simulink model "EngineModel_scaled_27_7_2016_with_new_maps"  (R2021a)
settings: Solver=ode4  StartTime=0.0  StopTime=30  FixedStep=0.2  RelTol=1e-3  EnableMultiTasking=on
values from neighbouring files (symbols this model uses):
  Fanmap_2 = [1 1 1 1 1 1 1 1 1 1 275.724 325.4224 ... (330 elements, 10x3x11)]    [enginemaps2.mat]
  HPCompmap_2 = [1 1 1 1 1 1 1 1 1 1 32.390865 37.6623195 ... (330 elements, 10x3x11)]    [enginemaps2.mat]
  HPTurbinemap_2 = [0.24979968 0.24979968 0.24979968 0.24979968 0.24979968 0.24979968 0.24979968 0.24979968 0.24979968 0.24979968 0.004250667 0.005047667 ... (330 elements, 10x3x11)]    [enginemaps2.mat]
  LPCompmap_2 = [1 1 1 1 1 1 1 1 1 1 34.17260994 40.23277722 ... (330 elements, 10x3x11)]    [enginemaps2.mat]
  LPTurbinemap_2 = [0.665969797 0.665969797 0.665969797 0.665969797 0.665969797 0.665969797 0.665969797 0.665969797 0.00912 0.013173333 0.015706667 0.01672 ... (264 elements, 8x3x11)]    [enginemaps2.mat]
undefined symbols (not defined in the file or in its folder): Adiabatic_compression_fan, Adiabatic_compression_HPC, Adiabatic_compression_LPC, coldnozzle, compression_ram, cond_f2, D, datatables, hotnozzle, HPT1, if_Nth, if_Ntl, if_Z, LPT, performance1, thermo_combustor, turbo
libraries: dspmtrx3 x10, aerolibatmos2 x8, dspsigattribs x3, dspsolvers x2, dspfactors x1
(part 1 of 14)
settings Model: Creator=BES  LastModifiedBy=PhD
settings SolverCC: ZeroCrossAlgorithm=Adaptive  AlgebraicLoopSolver=TrustRegion
settings DataIOCC: InitialState=load('enginemaps1.mat')  SaveFormat=Array  ReturnWorkspaceOutputs=off
settings OptimizationCC: LifeSpan=inf
settings DebuggingCC: UnderspecifiedInitializationDetection=Classic  MergeDetectMultiDrivingBlocksExec=none  SolverPrmCheckMsg=warning  StateNameClashWarn=warning  SFUnexpectedBacktrackingDiag=warning  SFNoUnconditionalDefaultTransitionDiag=warning  SFExecutionAtInitializationDiag=none  SFMachineParentedDataDiag=warning  ArithmeticOperatorsInVariantConditions=warning
settings HardwareCC: ProdBitPerPointer=32  ProdBitPerSizeT=32  ProdBitPerPtrDiffT=32  ProdLargestAtomicFloat=None  ProdIntDivRoundTo=Undefined  ProdEndianess=Unspecified  ProdWordSize=32  ProdHWDeviceType=32-bit Generic
settings ModelReferenceCC: PropagateSignalLabelsOutOfModel=off
settings SFSimCC: SimUseLocalCustomCode=off  CustomCodeUndefinedFunction=UseInterfaceOnly
settings RTWCC: RTWUseLocalCustomCode=off
settings CodeAppCC: StateflowObjectComments=on
settings GRTTargetCC: TargetLangStandard=C89/C90 (ANSI)
settings ConfigComp: CovMetricSettings=dw  CovSaveCumulativeToWorkspaceVar=on  CovSaveSingleToWorkspaceVar=on  CovExternalEMLEnable=off
settings SimscapeCC: SimscapeNormalizeSystem=off
settings ConfigurationSet: Description=SimMechanics 2G

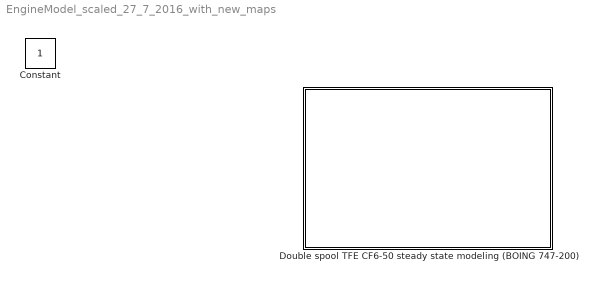
== system EngineModel_scaled_27_7_2016_with_new_maps ==
  Double spool TFE CF6-50 steady state modeling (BOING 747-200) : Subsystem
      mask Display: image('b747.jpg')
  Constant : Constant  IOType=siggen

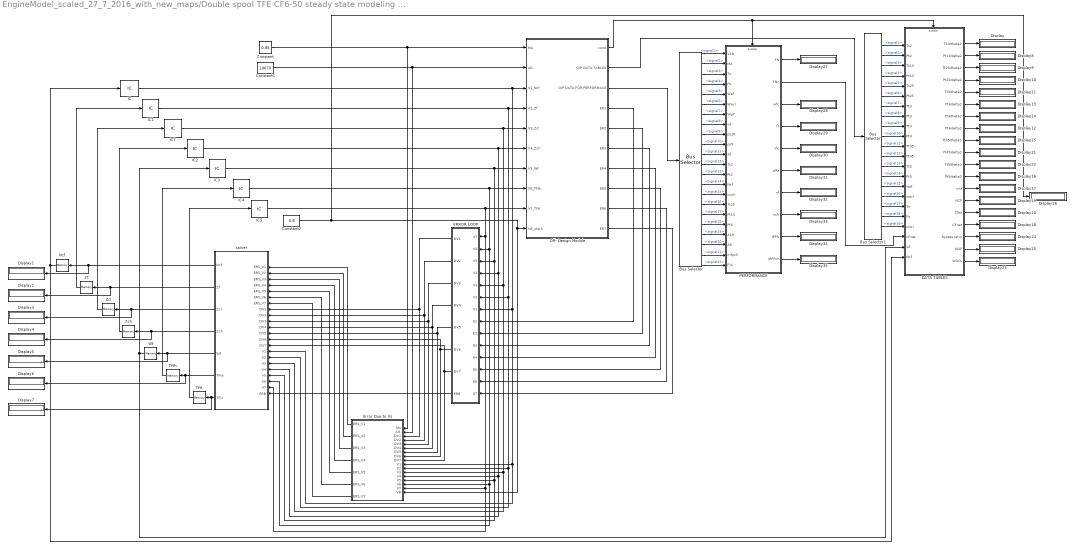
== system EngineModel_scaled_27_7_2016_with_new_maps/Double spool TFE CF6-50 steady state modeling (BOING 747-200) ==
  Bus Selector : BusSelector  OutputSignals=signal1,signal2,signal3,signal4,signal5,signal6,signal7,signal8,signal9,signal10,signal11,signal12,signal13,signal14,signal15,signal16,signal17,signal18,signal19,signal20,signal21,signal22
  Bus Selector1 : BusSelector  OutputSignals=signal1,signal2,signal3,signal4,signal5,signal6,signal7,signal8,signal9,signal10,signal11,signal12,signal13,signal14,signal15,signal16,signal17,signal18,signal19
  Constant : Constant  Value=0.85
  Constant1 : Constant  Value=10670
  Constant2 : Constant  Value=0.8  VectorParams1D=off
  DATA TABLES : Subsystem
  Display{,1..35} (36 alike) : Display
  "ERROR LOOP " : Subsystem
  Error Due to Vs : Subsystem
  IC : InitialCondition
  IC1 : InitialCondition  Value=0.83333
  IC2 : InitialCondition  Value=0.83333
  IC3 : InitialCondition  Value=0.89
  IC4 : InitialCondition  Value=156
  IC5 : InitialCondition  Value=674
  IC7 : InitialCondition  Value=0.83333
  Ncf : Memory  InitialCondition=1
  Off- Design Module : Subsystem
  PERFORMANCE : Subsystem
  TFth : Memory  InitialCondition=156
  TFtl : Memory  InitialCondition=674
  Wf : Memory  InitialCondition=0.89
  Zch : Memory  InitialCondition=0.83333
  Zcl : Memory  InitialCondition=0.83333
  Zf : Memory  InitialCondition=0.83333
  solver : Subsystem
  wires:
  Constant/1 -> Error Due to Vs/1(Mo), Off- Design Module/1(Mo)
  Constant1/1 -> Error Due to Vs/2(Alt.), Off- Design Module/2(Alt.)
  "ERROR LOOP "/1(DV1) -> solver/8(DV1), Error Due to Vs/3(DV1)
  "ERROR LOOP "/2(DV2) -> solver/9(DV2), Error Due to Vs/4(DV2)
  "ERROR LOOP "/3(DV3) -> solver/10(DV3), Error Due to Vs/5(DV3)
  "ERROR LOOP "/4(DV4) -> solver/11(DV4), Error Due to Vs/6(DV4)
  "ERROR LOOP "/5(DV5) -> solver/12(DV5), Error Due to Vs/7(DV5)
  "ERROR LOOP "/6(DV6) -> solver/13(DV6), Error Due to Vs/8(DV6)
  "ERROR LOOP "/7(DV7) -> solver/14(DV7), Error Due to Vs/9(DV7)
  solver/1(Ncf) -> Display1/1, Ncf/1
  solver/2(Zf) -> Zf/1, Display2/1
  solver/3(Zcl) -> Display3/1, Zcl/1
  solver/4(Zch) -> Display4/1, Zch/1
  solver/5(Wf) -> Display5/1, Wf/1
  solver/6(TFth) -> Display6/1, TFth/1
  solver/7(TFtl) -> Display7/1, TFtl/1
  Off- Design Module/4(ER1) -> "ERROR LOOP "/8(E1)
  Off- Design Module/5(ER2) -> "ERROR LOOP "/9(E2)
  Off- Design Module/6(ER3) -> "ERROR LOOP "/10(E3)
  Off- Design Module/7(ER4) -> "ERROR LOOP "/11(E4)
  Off- Design Module/8(ER5) -> "ERROR LOOP "/12(E5)
  Off- Design Module/9(ER6) -> "ERROR LOOP "/13(E6)
  Off- Design Module/10(ER7) -> "ERROR LOOP "/14(E7)
  "ERROR LOOP "/8(ERB) -> solver/22(ERB)
  Error Due to Vs/1(ERS_V1) -> solver/1(ERS_V1)
  Error Due to Vs/2(ERS_V2) -> solver/2(ERS_V2)
  Error Due to Vs/3(ERS_V3) -> solver/3(ERS_V3)
  Error Due to Vs/4(ERS_V4) -> solver/4(ERS_V4)
  Error Due to Vs/5(ERS_V5) -> solver/5(ERS_V5)
  Error Due to Vs/6(ERS_V6) -> solver/6(ERS_V6)
  Error Due to Vs/7(ERS_V7) -> solver/7(ERS_V7)
  IC/1 -> Off- Design Module/3(V1_Ncf), Error Due to Vs/10(V1), solver/15(V1), "ERROR LOOP "/7(V1)
  IC1/1 -> Off- Design Module/4(V2_Zf), solver/16(V2), Error Due to Vs/11(V2), "ERROR LOOP "/6(V2)
  IC7/1 -> Off- Design Module/5(V3_Zcl), "ERROR LOOP "/5(V3), solver/17(V3), Error Due to Vs/12(V3)
  IC2/1 -> solver/18(V4), Error Due to Vs/13(V4), "ERROR LOOP "/4(V4), Off- Design Module/6(V4_Zch)
  IC3/1 -> solver/19(V5), Error Due to Vs/14(V5), "ERROR LOOP "/3(V5), Off- Design Module/7(V5_Wf)
  IC4/1 -> solver/20(V6), Error Due to Vs/15(V6), "ERROR LOOP "/2(V6), Off- Design Module/8(V6_TFth)
  IC5/1 -> Off- Design Module/9(V7_TFtl), solver/21(V7), Error Due to Vs/16(V7), "ERROR LOOP "/1(V7)
  Constant2/1 -> Display26/1, Error Due to Vs/17(VB), Off- Design Module/10(VB_cNch)
  Off- Design Module/3(O/P DATA FOR PERFORMACE) -> Bus Selector/1
  Off- Design Module/1(cond) -> DATA TABLES/Enable, PERFORMANCE/Enable
  Bus Selector/20 -> PERFORMANCE/20(A9)  "<signal20>"
  Bus Selector/19 -> PERFORMANCE/19(A19)  "<signal19>"
  Bus Selector/18 -> PERFORMANCE/18(Pt5)  "<signal18>"
  Bus Selector/17 -> PERFORMANCE/17(Pt13)  "<signal17>"
  Bus Selector/16 -> PERFORMANCE/16(Tt25)  "<signal16>"
  Bus Selector/15 -> PERFORMANCE/15(cnch)  "<signal15>"
  Bus Selector/14 -> PERFORMANCE/14(Ncf)  "<signal14>"
  Bus Selector/13 -> PERFORMANCE/13(Pt2)  "<signal13>"
  Bus Selector/12 -> PERFORMANCE/12(Tt2)  "<signal12>"
  Bus Selector/11 -> PERFORMANCE/11(wf)  "<signal11>"
  Bus Selector/10 -> PERFORMANCE/10(ps9)  "<signal10>"
  Bus Selector/9 -> PERFORMANCE/9(ps10)  "<signal9>"
  Bus Selector/8 -> PERFORMANCE/8(v9)  "<signal8>"
  Bus Selector/7 -> PERFORMANCE/7(Wg7)  "<signal7>"
  Bus Selector/6 -> PERFORMANCE/6(Wacl)  "<signal6>"
  Bus Selector/5 -> PERFORMANCE/5(Waf)  "<signal5>"
  Bus Selector/4 -> PERFORMANCE/4(Po)  "<signal4>"
  Bus Selector/3 -> PERFORMANCE/3(To)  "<signal3>"
  Bus Selector/2 -> PERFORMANCE/2(Mo)  "<signal2>"
  Bus Selector/1 -> PERFORMANCE/1(V19)  "<signal1>"
  TFtl/1 -> IC5/1
  TFth/1 -> IC4/1
  Wf/1 -> DATA TABLES/21(wf), IC3/1
  Zch/1 -> IC2/1
  Zcl/1 -> IC7/1
  Zf/1 -> IC1/1
  Ncf/1 -> DATA TABLES/22(Ncf), IC/1
  Off- Design Module/2(O/P DATA TABLES) -> Bus Selector1/1
  Bus Selector1/1 -> DATA TABLES/1(Tt2)  "<signal1>"
  Bus Selector1/2 -> DATA TABLES/2(Pt2)  "<signal2>"
  Bus Selector1/3 -> DATA TABLES/3(Tt13)  "<signal3>"
  Bus Selector1/4 -> DATA TABLES/4(Pt13)  "<signal4>"
  Bus Selector1/5 -> DATA TABLES/5(Tt25)  "<signal5>"
  Bus Selector1/6 -> DATA TABLES/6(Pt25)  "<signal6>"
  Bus Selector1/7 -> DATA TABLES/7(Tt3)  "<signal7>"
  Bus Selector1/8 -> DATA TABLES/8(Pt3)  "<signal8>"
  Bus Selector1/9 -> DATA TABLES/9(Tt4)  "<signal9>"
  Bus Selector1/10 -> DATA TABLES/10(Pt4)  "<signal10>"
  Bus Selector1/11 -> DATA TABLES/11(Tt45)  "<signal11>"
  Bus Selector1/12 -> DATA TABLES/12(Pt45)  "<signal12>"
  Bus Selector1/13 -> DATA TABLES/13(Tt5)  "<signal13>"
  Bus Selector1/14 -> DATA TABLES/14(Pt5)  "<signal14>"
  Bus Selector1/15 -> DATA TABLES/15(waf)  "<signal15>"
  Bus Selector1/16 -> DATA TABLES/16(wacl)  "<signal16>"
  Bus Selector1/17 -> DATA TABLES/17(To)  "<signal17>"
  Bus Selector1/18 -> DATA TABLES/18(Po)  "<signal18>"
  Bus Selector1/19 -> DATA TABLES/19(cNcl)  "<signal19>"
  PERFORMANCE/2(FNc) -> DATA TABLES/20(cFnet)
  DATA TABLES/1(T13/theta2) -> Display/1
  DATA TABLES/2(Pt13/delta2) -> Display8/1
  DATA TABLES/3(Tt25/theta2) -> Display9/1
  DATA TABLES/4(Pt25/delta2) -> Display10/1
  DATA TABLES/5(Tt3/theta2) -> Display11/1
  DATA TABLES/6(Pt3/delta2) -> Display13/1
  DATA TABLES/7(Tt4/theta2) -> Display14/1
  DATA TABLES/8(Pt4/delta2) -> Display12/1
  DATA TABLES/9(Tt45/theta2) -> Display15/1
  DATA TABLES/10(Pt45/delta2) -> Display21/1
  DATA TABLES/11(Tt5/theta2) -> Display22/1
  DATA TABLES/12(Pt5/delta2) -> Display16/1
  DATA TABLES/13(cwf) -> Display17/1
  DATA TABLES/14(NCF) -> Display19/1
  DATA TABLES/15(CNcl) -> Display20/1
  DATA TABLES/16(CFnet) -> Display18/1
  DATA TABLES/17(bypass ratio) -> Display24/1
  DATA TABLES/18(WAF) -> Display25/1
  DATA TABLES/19(WACL) -> Display23/1
  Bus Selector/21 -> PERFORMANCE/21(mfpch)  "<signal21>"
  Bus Selector/22 -> PERFORMANCE/22(F/A)  "<signal22>"
  PERFORMANCE/1(FN) -> Display27/1
  PERFORMANCE/3(wfc) -> Display28/1
  PERFORMANCE/4(fs) -> Display29/1
  PERFORMANCE/5(sfc) -> Display30/1
  PERFORMANCE/6(alfa) -> Display31/1
  PERFORMANCE/7(nf) -> Display32/1
  PERFORMANCE/8(nch) -> Display33/1
  PERFORMANCE/9(IEPR) -> Display34/1
  PERFORMANCE/10(MFPch) -> Display35/1

== system EngineModel_scaled_27_7_2016_with_new_maps/Double spool TFE CF6-50 steady state modeling (BOING 747-200)/DATA TABLES ==
  Tt2 : Inport
  Pt2 : Inport  Port=2
  Tt13 : Inport  Port=3
  Pt13 : Inport  Port=4
  Tt25 : Inport  Port=5
  Pt25 : Inport  Port=6
  Tt3 : Inport  Port=7
  Pt3 : Inport  Port=8
  Tt4 : Inport  Port=9
  Pt4 : Inport  Port=10
  Tt45 : Inport  Port=11
  Pt45 : Inport  Port=12
  Tt5 : Inport  Port=13
  Pt5 : Inport  Port=14
  waf : Inport  Port=15
  wacl : Inport  Port=16
  To : Inport  Port=17
  Po : Inport  Port=18
  cNcl : Inport  Port=19
  cFnet : Inport  Port=20
  wf : Inport  Port=21
  Ncf : Inport  Port=22
  Enable : EnablePort  StatesWhenEnabling=reset
  Bus Creator : BusCreator  Inputs=19
  Demux : Demux  Outputs=19
      settings: DisplayOption=none
  Interpreted MATLAB Function : MATLABFcn  MATLABFcn=datatables (u(1),u(2),u(3),u(4),u(5),u(6),u(7),u(8),u(9),u(10),u(11),u(12),u(13),u(14),u(15),u(16),u(17),u(18),u(19),u(20),u(21),u(22))  OutputDimensions=19
  Mux : Mux  Inputs=22
      settings: DisplayOption=signals
  To File : ToFile  Filename=datatable.mat  MatrixName=bes
  T13/theta2 : Outport
  Pt13/delta2 : Outport  Port=2
  Tt25/theta2 : Outport  Port=3
  Pt25/delta2 : Outport  Port=4
  Tt3/theta2 : Outport  Port=5
  Pt3/delta2 : Outport  Port=6
  Tt4/theta2 : Outport  Port=7
  Pt4/delta2 : Outport  Port=8
  Tt45/theta2 : Outport  Port=9
  Pt45/delta2 : Outport  Port=10
  Tt5/theta2 : Outport  Port=11
  Pt5/delta2 : Outport  Port=12
  cwf : Outport  Port=13
  NCF : Outport  Port=14
  CNcl : Outport  Port=15
  CFnet : Outport  Port=16
  bypass ratio : Outport  Port=17
  WAF : Outport  Port=18
  WACL : Outport  Port=19
  wires:
  Pt5/1 -> Mux/14
  Tt5/1 -> Mux/13
  Pt45/1 -> Mux/12
  Tt45/1 -> Mux/11
  Pt4/1 -> Mux/10
  Pt3/1 -> Mux/8
  Tt3/1 -> Mux/7
  Pt25/1 -> Mux/6
  Tt25/1 -> Mux/5
  Pt13/1 -> Mux/4
  Tt13/1 -> Mux/3
  Pt2/1 -> Mux/2
  Tt2/1 -> Mux/1
  Interpreted MATLAB Function/1 -> Demux/1
  Mux/1 -> Interpreted MATLAB Function/1
  waf/1 -> Mux/15
  cNcl/1 -> Mux/19
  wacl/1 -> Mux/16
  To/1 -> Mux/17
  Po/1 -> Mux/18
  cFnet/1 -> Mux/20
  wf/1 -> Mux/21
  Ncf/1 -> Mux/22
  Demux/1 -> Bus Creator/1, T13/theta2/1
  Demux/4 -> Bus Creator/4, Pt25/delta2/1
  Demux/5 -> Bus Creator/5, Tt3/theta2/1
  Demux/6 -> Bus Creator/6, Pt3/delta2/1
  Demux/7 -> Bus Creator/7, Tt4/theta2/1
  Demux/8 -> Bus Creator/8, Pt4/delta2/1
  Demux/9 -> Bus Creator/9, Tt45/theta2/1
  Demux/11 -> Bus Creator/11, Tt5/theta2/1
  Demux/12 -> Bus Creator/12, Pt5/delta2/1
  Demux/13 -> Bus Creator/13, cwf/1
  Demux/14 -> Bus Creator/14, NCF/1
  Demux/15 -> Bus Creator/15, CNcl/1
  Demux/16 -> Bus Creator/16, CFnet/1
  Demux/17 -> Bus Creator/17, bypass ratio/1
  Demux/18 -> Bus Creator/18, WAF/1
  Demux/19 -> Bus Creator/19, WACL/1
  Demux/2 -> Bus Creator/2, Pt13/delta2/1
  Bus Creator/1 -> To File/1
  Demux/3 -> Bus Creator/3, Tt25/theta2/1
  Demux/10 -> Bus Creator/10, Pt45/delta2/1
  Tt4/1 -> Mux/9

== system EngineModel_scaled_27_7_2016_with_new_maps/Double spool TFE CF6-50 steady state modeling (BOING 747-200)/ERROR LOOP  ==
  V7 : Inport
  V6 : Inport  Port=2
  V5 : Inport  Port=3
  V4 : Inport  Port=4
  V3 : Inport  Port=5
  V2 : Inport  Port=6
  V1 : Inport  Port=7
  E1 : Inport  Port=8
  E2 : Inport  Port=9
  E3 : Inport  Port=10
  E4 : Inport  Port=11
  E5 : Inport  Port=12
  E6 : Inport  Port=13
  E7 : Inport  Port=14
  Constant : Constant  Value=0.005
  Constant1 : Constant  Value=100
  Display1 : Display
  Divide : Product  Inputs=*/
  Divide1 : Product  Inputs=*/
  Product{,1..6} (7 alike) : Product
  Vector Concatenate : Concatenate  NumInputs=7  Mode=Multidimensional array
  DV1 : Outport
  DV2 : Outport  Port=2
  DV3 : Outport  Port=3
  DV4 : Outport  Port=4
  DV5 : Outport  Port=5
  DV6 : Outport  Port=6
  DV7 : Outport  Port=7
  ERB : Outport  Port=8
  wires:
  Constant/1 -> Product6/1, Product5/1, Product4/1, Product3/1, Product2/1, Product1/1, Product/1
  V5/1 -> Product2/2
  V1/1 -> Product6/2
  V2/1 -> Product5/2
  V3/1 -> Product4/2
  V4/1 -> Product3/2
  Product3/1 -> DV4/1
  Product4/1 -> DV3/1
  Product5/1 -> DV2/1
  Product6/1 -> DV1/1
  E1/1 -> Vector Concatenate/1
  E2/1 -> Vector Concatenate/2
  E3/1 -> Vector Concatenate/3
  E4/1 -> Vector Concatenate/4
  E5/1 -> Vector Concatenate/5
  E6/1 -> Vector Concatenate/6
  E7/1 -> Vector Concatenate/7
  Vector Concatenate/1 -> Display1/1, ERB/1
  Product2/1 -> DV5/1
  Product/1 -> DV7/1
  Product1/1 -> DV6/1
  V7/1 -> Divide/1
  Constant1/1 -> Divide1/2, Divide/2
  Divide/1 -> Product/2
  V6/1 -> Divide1/1
  Divide1/1 -> Product1/2

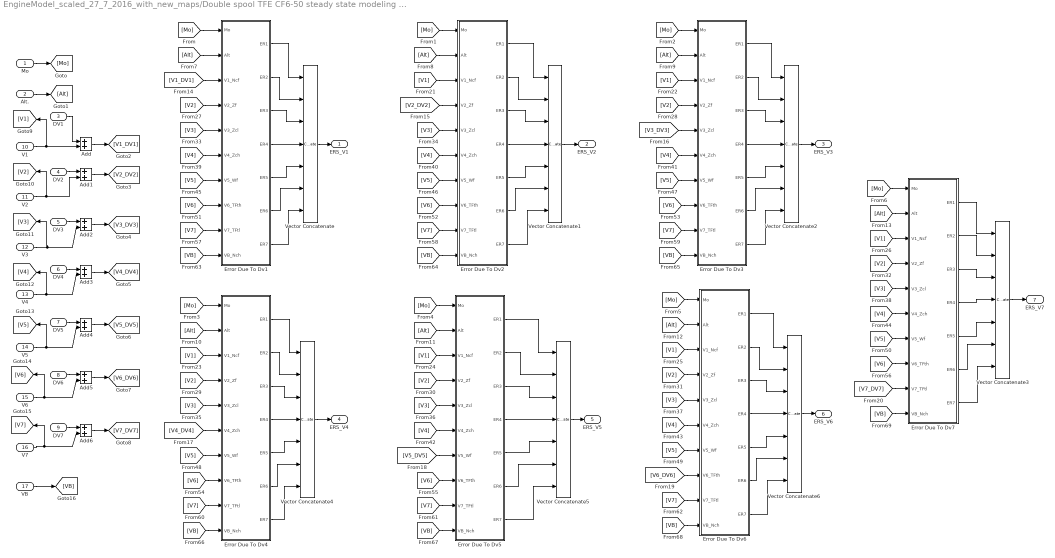
== system EngineModel_scaled_27_7_2016_with_new_maps/Double spool TFE CF6-50 steady state modeling (BOING 747-200)/Error Due to Vs ==
  Mo : Inport
  Alt. : Inport  Port=2
  DV1 : Inport  Port=3
  DV2 : Inport  Port=4
  DV3 : Inport  Port=5
  DV4 : Inport  Port=6
  DV5 : Inport  Port=7
  DV6 : Inport  Port=8
  DV7 : Inport  Port=9
  V1 : Inport  Port=10
  V2 : Inport  Port=11
  V3 : Inport  Port=12
  V4 : Inport  Port=13
  V5 : Inport  Port=14
  V6 : Inport  Port=15
  V7 : Inport  Port=16
  VB : Inport  Port=17
  Add{,1..6} (7 alike) : Sum
  Error Due To Dv1 : Subsystem
  Error Due To Dv2 : Subsystem
  Error Due To Dv3 : Subsystem
  Error Due To Dv4 : Subsystem
  Error Due To Dv5 : Subsystem
  Error Due To Dv6 : Subsystem
  Error Due To Dv7 : Subsystem
  Vector Concatenate{,1..6} (7 alike) : Concatenate  NumInputs=7
  ERS_V1 : Outport
  ERS_V2 : Outport  Port=2
  ERS_V3 : Outport  Port=3
  ERS_V4 : Outport  Port=4
  ERS_V5 : Outport  Port=5
  ERS_V6 : Outport  Port=6
  ERS_V7 : Outport  Port=7
  wires:
  Vector Concatenate/1 -> ERS_V1/1
  Vector Concatenate1/1 -> ERS_V2/1
  Vector Concatenate2/1 -> ERS_V3/1
  Vector Concatenate4/1 -> ERS_V4/1
  Vector Concatenate5/1 -> ERS_V5/1
  Vector Concatenate6/1 -> ERS_V6/1
  Vector Concatenate3/1 -> ERS_V7/1
  Error Due To Dv1/1(ER1) -> Vector Concatenate/1
  Error Due To Dv1/2(ER2) -> Vector Concatenate/2
  Error Due To Dv1/3(ER3) -> Vector Concatenate/3
  Error Due To Dv1/4(ER4) -> Vector Concatenate/4
  Error Due To Dv1/5(ER5) -> Vector Concatenate/5
  Error Due To Dv1/6(ER6) -> Vector Concatenate/6
  Error Due To Dv1/7(ER7) -> Vector Concatenate/7
  Error Due To Dv2/4(ER4) -> Vector Concatenate1/4
  Error Due To Dv2/1(ER1) -> Vector Concatenate1/1
  Error Due To Dv2/3(ER3) -> Vector Concatenate1/3
  Error Due To Dv2/2(ER2) -> Vector Concatenate1/2
  Error Due To Dv2/7(ER7) -> Vector Concatenate1/7
  Error Due To Dv2/5(ER5) -> Vector Concatenate1/5
  Error Due To Dv2/6(ER6) -> Vector Concatenate1/6
  Error Due To Dv3/4(ER4) -> Vector Concatenate2/4
  Error Due To Dv3/1(ER1) -> Vector Concatenate2/1
  Error Due To Dv3/7(ER7) -> Vector Concatenate2/7
  Error Due To Dv3/2(ER2) -> Vector Concatenate2/2
  Error Due To Dv3/3(ER3) -> Vector Concatenate2/3
  Error Due To Dv3/6(ER6) -> Vector Concatenate2/6
  Error Due To Dv3/5(ER5) -> Vector Concatenate2/5
  Error Due To Dv4/1(ER1) -> Vector Concatenate4/1
  Error Due To Dv4/4(ER4) -> Vector Concatenate4/4
  Error Due To Dv4/3(ER3) -> Vector Concatenate4/3
  Error Due To Dv4/2(ER2) -> Vector Concatenate4/2
  Error Due To Dv4/5(ER5) -> Vector Concatenate4/5
  Error Due To Dv4/7(ER7) -> Vector Concatenate4/7
  Error Due To Dv4/6(ER6) -> Vector Concatenate4/6
  Error Due To Dv5/1(ER1) -> Vector Concatenate5/1
  Error Due To Dv5/2(ER2) -> Vector Concatenate5/2
  Error Due To Dv5/3(ER3) -> Vector Concatenate5/3
  Error Due To Dv5/4(ER4) -> Vector Concatenate5/4
  Error Due To Dv5/5(ER5) -> Vector Concatenate5/5
  Error Due To Dv5/6(ER6) -> Vector Concatenate5/6
  Error Due To Dv5/7(ER7) -> Vector Concatenate5/7
  Error Due To Dv6/4(ER4) -> Vector Concatenate6/4
  Error Due To Dv6/1(ER1) -> Vector Concatenate6/1
  Error Due To Dv6/2(ER2) -> Vector Concatenate6/2
  Error Due To Dv6/3(ER3) -> Vector Concatenate6/3
  Error Due To Dv6/5(ER5) -> Vector Concatenate6/5
  Error Due To Dv6/6(ER6) -> Vector Concatenate6/6
  Error Due To Dv6/7(ER7) -> Vector Concatenate6/7
  Error Due To Dv7/4(ER4) -> Vector Concatenate3/4
  Error Due To Dv7/1(ER1) -> Vector Concatenate3/1
  Error Due To Dv7/2(ER2) -> Vector Concatenate3/2
  Error Due To Dv7/3(ER3) -> Vector Concatenate3/3
  Error Due To Dv7/5(ER5) -> Vector Concatenate3/5
  Error Due To Dv7/6(ER6) -> Vector Concatenate3/6
  DV1/1 -> Add/1
  V1/1 -> [V1], Add/2
  DV2/1 -> Add1/1
  DV3/1 -> Add2/1
  DV4/1 -> Add3/1
  DV5/1 -> Add4/1
  DV6/1 -> Add5/1
  DV7/1 -> Add6/1
  Error Due To Dv7/7(ER7) -> Vector Concatenate3/7
  Mo/1 -> [Mo]
  [Mo] -> Error Due To Dv1/1(Mo)
  [Mo] -> Error Due To Dv2/1(Mo)
  [Mo] -> Error Due To Dv3/1(Mo)
  [Mo] -> Error Due To Dv4/1(Mo)
  [Mo] -> Error Due To Dv5/1(Mo)
  [Mo] -> Error Due To Dv6/1(Mo)
  [Mo] -> Error Due To Dv7/1(Mo)
  [Alt] -> Error Due To Dv1/2(Alt)
  Alt./1 -> [Alt]
  [Alt] -> Error Due To Dv2/2(Alt)
  [Alt] -> Error Due To Dv3/2(Alt)
  [Alt] -> Error Due To Dv4/2(Alt)
  [Alt] -> Error Due To Dv5/2(Alt)
  [Alt] -> Error Due To Dv6/2(Alt)
  [Alt] -> Error Due To Dv7/2(Alt)
  Add/1 -> [V1_DV1]
  Add1/1 -> [V2_DV2]
  Add2/1 -> [V3_DV3]
  Add3/1 -> [V4_DV4]
  Add4/1 -> [V5_DV5]
  Add5/1 -> [V6_DV6]
  Add6/1 -> [V7_DV7]
  [V1_DV1] -> Error Due To Dv1/3(V1_Ncf)
  [V2_DV2] -> Error Due To Dv2/4(V2_Zf)
  [V3_DV3] -> Error Due To Dv3/5(V3_Zcl)
  [V4_DV4] -> Error Due To Dv4/6(V4_Zch)
  [V5_DV5] -> Error Due To Dv5/7(V5_Wf)
  [V6_DV6] -> Error Due To Dv6/8(V6_TFth)
  [V7_DV7] -> Error Due To Dv7/9(V7_TFtl)
  V2/1 -> [V2], Add1/2
  V3/1 -> [V3], Add2/2
  V4/1 -> [V4], Add3/2
  V5/1 -> [V5], Add4/2
  V6/1 -> [V6], Add5/2
  V7/1 -> Add6/2, [V7]
  VB/1 -> [VB]
  [V1] -> Error Due To Dv2/3(V1_Ncf)
  [V1] -> Error Due To Dv3/3(V1_Ncf)
  [V1] -> Error Due To Dv4/3(V1_Ncf)
  [V1] -> Error Due To Dv5/3(V1_Ncf)
  [V1] -> Error Due To Dv6/3(V1_Ncf)
  [V1] -> Error Due To Dv7/3(V1_Ncf)
  [V2] -> Error Due To Dv1/4(V2_Zf)
  [V2] -> Error Due To Dv3/4(V2_Zf)
  [V2] -> Error Due To Dv4/4(V2_Zf)
  [V2] -> Error Due To Dv5/4(V2_Zf)
  [V2] -> Error Due To Dv6/4(V2_Zf)
  [V2] -> Error Due To Dv7/4(V2_Zf)
  [V3] -> Error Due To Dv1/5(V3_Zcl)
  [V3] -> Error Due To Dv2/5(V3_Zcl)
  [V3] -> Error Due To Dv4/5(V3_Zcl)
  [V3] -> Error Due To Dv5/5(V3_Zcl)
  [V3] -> Error Due To Dv6/5(V3_Zcl)
  [V3] -> Error Due To Dv7/5(V3_Zcl)
  [V4] -> Error Due To Dv1/6(V4_Zch)
  [V4] -> Error Due To Dv2/6(V4_Zch)
  [V4] -> Error Due To Dv3/6(V4_Zch)
  [V4] -> Error Due To Dv5/6(V4_Zch)
  [V4] -> Error Due To Dv6/6(V4_Zch)
  [V4] -> Error Due To Dv7/6(V4_Zch)
  [V5] -> Error Due To Dv1/7(V5_Wf)
  [V5] -> Error Due To Dv2/7(V5_Wf)
  [V5] -> Error Due To Dv3/7(V5_Wf)
  [V5] -> Error Due To Dv4/7(V5_Wf)
  [V5] -> Error Due To Dv6/7(V5_Wf)
  [V5] -> Error Due To Dv7/7(V5_Wf)
  [V6] -> Error Due To Dv1/8(V6_TFth)
  [V6] -> Error Due To Dv2/8(V6_TFth)
  [V6] -> Error Due To Dv3/8(V6_TFth)
  [V6] -> Error Due To Dv4/8(V6_TFth)
  [V6] -> Error Due To Dv5/8(V6_TFth)
  [V6] -> Error Due To Dv7/8(V6_TFth)
  [V7] -> Error Due To Dv1/9(V7_TFtl)
  [V7] -> Error Due To Dv2/9(V7_TFtl)
  [V7] -> Error Due To Dv3/9(V7_TFtl)
  [V7] -> Error Due To Dv4/9(V7_TFtl)
  [V7] -> Error Due To Dv5/9(V7_TFtl)
  [V7] -> Error Due To Dv6/9(V7_TFtl)
  [VB] -> Error Due To Dv1/10(VB_Nch)
  [VB] -> Error Due To Dv2/10(VB_Nch)
  [VB] -> Error Due To Dv3/10(VB_Nch)
  [VB] -> Error Due To Dv4/10(VB_Nch)
  [VB] -> Error Due To Dv5/10(VB_Nch)
  [VB] -> Error Due To Dv6/10(VB_Nch)
  [VB] -> Error Due To Dv7/10(VB_Nch)

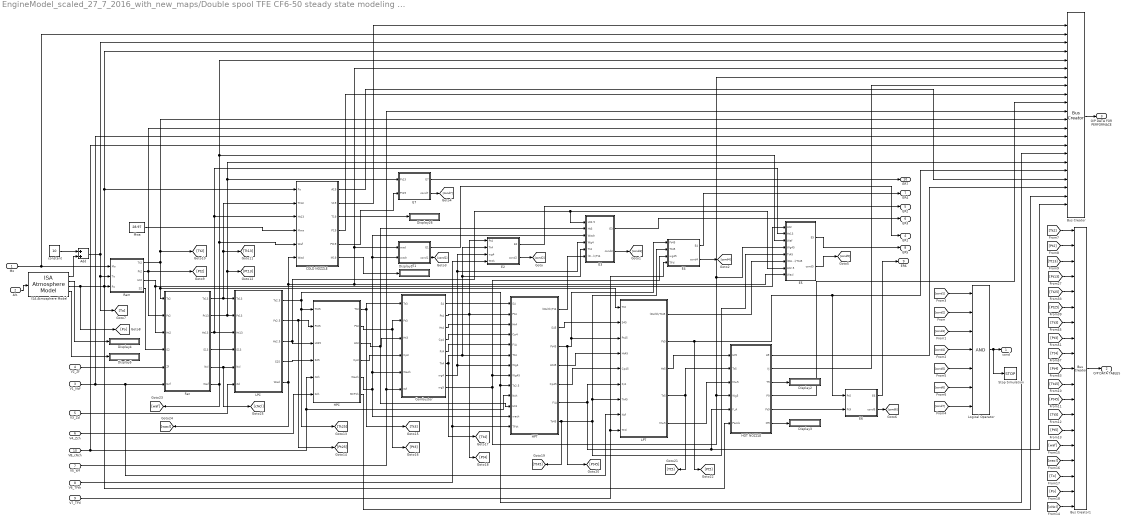
== system EngineModel_scaled_27_7_2016_with_new_maps/Double spool TFE CF6-50 steady state modeling (BOING 747-200)/Off- Design Module ==
  Mo : Inport
  Alt. : Inport  Port=2
  V1_Ncf : Inport  Port=3
  V2_Zf : Inport  Port=4
  V3_Zcl : Inport  Port=5
  V4_Zch : Inport  Port=6
  V5_Wf : Inport  Port=7
  V6_TFth : Inport  Port=8
  V7_TFtl : Inport  Port=9
  VB_cNch : Inport  Port=10
  Add : Sum
  Bus Creator : BusCreator  Inputs=22
  Bus Creator1 : BusCreator  Inputs=19
  COLD NOZZLE : Subsystem
  Combustor : Subsystem
  Display{1..5,26} (6 alike) : Display
  E1 : Subsystem
  E2 : Subsystem
  E3 : Subsystem
  E4 : Subsystem
  E5 : Subsystem  RequirementInfo={} %GIDa_96be69d7_9551_44df_92c2_7c0f27b37e06
  E6 : Subsystem
  E7 : Subsystem
  Fan : Subsystem
  HOT NOZZLE : Subsystem
  HPC : Subsystem
  HPT : Subsystem
  ISA Atmosphere Model : aerolibatmos2/ISA Atmosphere Model  custom=on  g=9.8  gamma=1.4  R=287  L=0.0065  h_trop=11000  h_strat=20000  rho0=1.225  P0=101325  T0=288  h0=0
  LPC : Subsystem
  LPT : Subsystem
  Logical Operator : Logic  Inputs=7  AllPortsSameDT=off  OutDataTypeStr=boolean
  Mwa : Constant  Value=28.97
  Ram : Subsystem
  Stop Simulation : Stop
  constant : Constant  Value=10
  cond : Outport
  O/P DATA TABLES : Outport  Port=2
  O/P DATA FOR PERFORMACE : Outport  Port=3
  ER1 : Outport  Port=4
  ER2 : Outport  Port=5
  ER3 : Outport  Port=6
  ER4 : Outport  Port=7
  ER5 : Outport  Port=8
  ER6 : Outport  Port=9
  ER7 : Outport  Port=10
  wires:
  Alt./1 -> ISA Atmosphere Model/1
  Mo/1 -> Bus Creator/2, Ram/1(Mo)
  Add/1 -> Bus Creator/3, [To], Ram/2(To)
  ISA Atmosphere Model/3 -> [Po], HOT NOZZLE/6(Pamb), Ram/3(Po), Bus Creator/4, COLD NOZZLE/1(Po)
  constant/1 -> Add/1
  Ram/1(Tt2) -> [Tt2], Bus Creator/12, Fan/1(Tt2), LPT/1(Tt2)
  Ram/2(Pt2) -> [Pt2], Bus Creator/13, Fan/2(Pt2)
  HPC/2(Pt3) -> Combustor/2(Pt3), [Pt3]
  HPC/3(Ht3) -> Combustor/3(Ht3), E3/2(Ht3), HPT/11(Ht3)
  Combustor/2(Pt4) -> [Pt4], HPT/2(Pt4), E2/1(Pt4)
  Combustor/4(Cp4) -> HPT/4(Cp4)
  Combustor/5(F/A) -> HPT/5(F/A)
  Combustor/6(Tt4) -> [Tt4], HPT/6(Tt4), E2/2(Tt4), E3/5(Tt4)
  LPT/3(Ht5) -> HOT NOZZLE/1(Ht5)
  LPT/4(Tt5) -> HOT NOZZLE/2(Tt5), [Tt5]
  V2_Zf/1 -> Fan/5(Zf)
  V1_Ncf/1 -> Bus Creator/14, LPT/8(Ncf), Fan/6(Ncf)
  V3_Zcl/1 -> LPC/6(Zcl)
  V4_Zch/1 -> HPC/6(Zch)
  VB_cNch/1 -> Bus Creator/15, HPC/5(Nch), HPT/10(Nch)
  V5_Wf/1 -> Bus Creator/11, Combustor/6(Wf)
  V6_TFth/1 -> E2/4(TFth), HPT/13(TFth)
  Combustor/7(wg4) -> E2/3(wg4), E3/4(Wg4), HPT/7(Wg4)
  LPT/5(Mw5) -> HOT NOZZLE/3(Mw5)
  Fan/3(Ht13) -> E5/2(Ht13), COLD NOZZLE/3(Ht13), LPC/3(Ht13)
  Mwa/1 -> COLD NOZZLE/4(Mwa)
  Fan/6(Waf) -> Bus Creator/5, E5/3(Waf), COLD NOZZLE/5(Waf), [waf]
  LPC/5(Wacl) -> COLD NOZZLE/6(Wacl), Bus Creator/6, E1/1(wacl), E5/8(Wacl), [wacl]
  COLD NOZZLE/5(Pt19) -> E7/2(Pt19)
  LPC/3(Ht2.5) -> E3/1(Ht2.5), E5/7(Ht2.5), HPC/3(Ht25)
  LPT/2(Pt5) -> [Pt5], Bus Creator/18, E6/1(Pt5)
  HOT NOZZLE/5(Pt9) -> E6/2(Pt9)
  LPT/1((DH)th/Tt45) -> E5/6((DH)tl/Tt45)
  Combustor/8(wg5) -> HPT/8(Wg45), E4/3(wg45), Bus Creator/7, E5/4(Wg45), HOT NOZZLE/4(Wg5)
  Combustor/3(Ht4) -> HPT/3(Ht4)
  Combustor/1(S4) -> HPT/1(S4)
  Ram/3(Ht2) -> Fan/3(Ht2), E5/1(Ht2)
  Ram/4(S2) -> Fan/4(S2)
  Fan/5(Ncl) -> [cNcl], LPC/5(Ncl)
  Fan/4(S13) -> LPC/4(S13)
  LPC/4(S25) -> HPC/4(S25)
  HPC/5(Wach) -> HPT/12(wach), E3/3(Wach), E1/2(wach), Combustor/5(Wach)
  HPT/2(S45) -> LPT/2(S45)
  HPT/3(Pt45) -> [Pt45], E4/1(Pt45), LPT/3(Pt45)
  HPT/4(Ht45) -> LPT/4(Ht45)
  HPT/5(Cp45) -> LPT/5(Cp45)
  HPT/7(Tt45) -> [Tt45], LPT/7(Tt45), E4/2(Tt45), E5/5(Tt45)
  HPT/6(F\A) -> LPT/6(F/A), Bus Creator/22, HOT NOZZLE/5(F_A)
  V7_TFtl/1 -> LPT/9(TFtl), E4/4(TFtl)
  HPT/1((DH)th/Tt4) -> E3/6((DH)th/Tt4)
  E6/1(E6) -> ER6/1
  E5/1(E5) -> ER5/1
  E4/1(E4) -> ER4/1
  E3/1(E3) -> ER3/1
  E2/1(E2) -> ER2/1
  E7/1(E7) -> ER7/1
  E1/1(E1) -> ER1/1
  HOT NOZZLE/2(Vj) -> Bus Creator/8
  COLD NOZZLE/4(P19) -> Bus Creator/9
  HOT NOZZLE/4(P9) -> Bus Creator/10
  ISA Atmosphere Model/1 -> Add/2
  COLD NOZZLE/1(A19) -> Bus Creator/19
  HOT NOZZLE/1(A9) -> Bus Creator/20
  COLD NOZZLE/2(V19) -> Bus Creator/1
  Bus Creator/1 -> O/P DATA FOR PERFORMACE/1
  E6/2(cond6) -> [cond6]
  E5/2(cond5) -> [cond5]
  E4/2(cond4) -> [cond4]
  E3/2(cond3) -> [cond3]
  E2/2(cond2) -> [cond2]
  E1/2(cond1) -> [cond1]
  E7/2("cond7 ") -> [cond7]
  [cond1] -> Logical Operator/1
  [cond2] -> Logical Operator/2
  [cond3] -> Logical Operator/3
  [cond4] -> Logical Operator/4
  [cond5] -> Logical Operator/5
  [cond6] -> Logical Operator/6
  [cond7] -> Logical Operator/7
  Logical Operator/1 -> Stop Simulation/1, cond/1
  HPC/4(Cp3) -> Combustor/4(Cp3)
  [Tt2] -> Bus Creator1/1
  [Pt2] -> Bus Creator1/2
  [Tt13] -> Bus Creator1/3
  [Pt13] -> Bus Creator1/4
  [Tt25] -> Bus Creator1/5
  [Pt25] -> Bus Creator1/6
  [Tt3] -> Bus Creator1/7
  [Pt3] -> Bus Creator1/8
  [Tt4] -> Bus Creator1/9
  [Pt4] -> Bus Creator1/10
  [Tt45] -> Bus Creator1/11
  [Pt45] -> Bus Creator1/12
  [Tt5] -> Bus Creator1/13
  [Pt5] -> Bus Creator1/14
  [waf] -> Bus Creator1/15
  [wacl] -> Bus Creator1/16
  [To] -> Bus Creator1/17
  [Po] -> Bus Creator1/18
  Fan/1(Tt13) -> LPC/1(Tt13), [Tt13], COLD NOZZLE/2(Tt13)
  Fan/2(Pt13) -> [Pt13], Bus Creator/17, E7/1(Pt13), LPC/2(Pt13)
  LPC/1(Tt2.5) -> HPT/9(Tt2.5), Bus Creator/16, [Tt25], HPC/1(Tt25)
  LPC/2(Pt2.5) -> [Pt25], HPC/2(Pt25)
  HPC/1(Tt3) -> [Tt3], Combustor/1(Tt3)
  Bus Creator1/1 -> O/P DATA TABLES/1
  [cNcl] -> Bus Creator1/19
  HPC/6(MFPch) -> Bus Creator/21
  COLD NOZZLE/3(T19) -> Display26/1
  COLD NOZZLE/6(M19) -> Display1/1
  HOT NOZZLE/3(T9) -> Display2/1
  HOT NOZZLE/6(M9) -> Display3/1
  ISA Atmosphere Model/2 -> Display4/1
  ISA Atmosphere Model/4 -> Display5/1

== system EngineModel_scaled_27_7_2016_with_new_maps/Double spool TFE CF6-50 steady state modeling (BOING 747-200)/PERFORMANCE ==
  V19 : Inport
  Mo : Inport  Port=2
  To : Inport  Port=3
  Po : Inport  Port=4
  Waf : Inport  Port=5
  Wacl : Inport  Port=6
  Wg7 : Inport  Port=7
  v9 : Inport  Port=8
  ps10 : Inport  Port=9
  ps9 : Inport  Port=10
  wf : Inport  Port=11
  Tt2 : Inport  Port=12
  Pt2 : Inport  Port=13
  Ncf : Inport  Port=14
  cnch : Inport  Port=15
  Tt25 : Inport  Port=16
  Pt13 : Inport  Port=17
  Pt5 : Inport  Port=18
  A19 : Inport  Port=19
  A9 : Inport  Port=20
  mfpch : Inport  Port=21
  F/A : Inport  Port=22
  Enable : EnablePort  StatesWhenEnabling=reset
  Bus Creator : BusCreator  Inputs=6
  Demux : Demux  Outputs=10
      settings: DisplayOption=none
  Interpreted MATLAB Function : MATLABFcn  MATLABFcn=performance1 (u(1),u(2),u(3),u(4),u(5),u(6),u(7),u(8),u(9),u(10),u(11),u(12),u(13),u(14),u(15),u(16),u(17),u(18),u(19),u(20),u(21),u(22))  OutputDimensions=10
  Mux : Mux  Inputs=22
      settings: DisplayOption=signals
  To File : ToFile  Filename=datatable1.mat  MatrixName=bes1
  FN : Outport
  FNc : Outport  Port=2
  wfc : Outport  Port=3
  fs : Outport  Port=4
  sfc : Outport  Port=5
  alfa : Outport  Port=6
  nf : Outport  Port=7
  nch : Outport  Port=8
  IEPR : Outport  Port=9
  MFPch : Outport  Port=10
  wires:
  Mux/1 -> Interpreted MATLAB Function/1
  Interpreted MATLAB Function/1 -> Demux/1
  Demux/1 -> FN/1
  Demux/2 -> FNc/1
  Demux/3 -> wfc/1
  Demux/4 -> Bus Creator/1, fs/1
  Demux/5 -> Bus Creator/2, sfc/1
  Demux/6 -> alfa/1
  Demux/7 -> Bus Creator/3, nf/1
  Demux/8 -> Bus Creator/4, nch/1
  Demux/9 -> Bus Creator/5, IEPR/1
  V19/1 -> Mux/1
  Mo/1 -> Mux/2
  To/1 -> Mux/3
  Po/1 -> Mux/4
  Waf/1 -> Mux/5
  Wacl/1 -> Mux/6
  Wg7/1 -> Mux/7
  v9/1 -> Mux/8
  ps10/1 -> Mux/9
  ps9/1 -> Mux/10
  wf/1 -> Mux/11
  Tt2/1 -> Mux/12
  Pt2/1 -> Mux/13
  Ncf/1 -> Mux/14
  cnch/1 -> Mux/15
  Tt25/1 -> Mux/16
  Pt13/1 -> Mux/17
  Pt5/1 -> Mux/18
  A19/1 -> Mux/19
  A9/1 -> Mux/20
  Bus Creator/1 -> To File/1
  mfpch/1 -> Mux/21
  Demux/10 -> Bus Creator/6, MFPch/1
  F/A/1 -> Mux/22

== system EngineModel_scaled_27_7_2016_with_new_maps/Double spool TFE CF6-50 steady state modeling (BOING 747-200)/solver ==
  ERS_V1 : Inport
  ERS_V2 : Inport  Port=2
  ERS_V3 : Inport  Port=3
  ERS_V4 : Inport  Port=4
  ERS_V5 : Inport  Port=5
  ERS_V6 : Inport  Port=6
  ERS_V7 : Inport  Port=7
  DV1 : Inport  Port=8
  DV2 : Inport  Port=9
  DV3 : Inport  Port=10
  DV4 : Inport  Port=11
  DV5 : Inport  Port=12
  DV6 : Inport  Port=13
  DV7 : Inport  Port=14
  V1 : Inport  Port=15
  V2 : Inport  Port=16
  V3 : Inport  Port=17
  V4 : Inport  Port=18
  V5 : Inport  Port=19
  V6 : Inport  Port=20
  V7 : Inport  Port=21
  ERB : Inport  Port=22
  " LU Inverse" : Subsystem  AncestorBlock=dspinverses/ LU Inverse  mask(LU Inverse){}
      mask help: Matrix inverse using LU factorization.
      mask Help: eval('blocksethelp');
      mask Display:
      | text(0.25,0.85,'General')
      | text(0.25,0.70,'Inverse')
      | text(0.35,0.25,'(LU)')
  Add{,1..6} (7 alike) : Sum
  Constant : Constant  Value=0.1
  Constant1 : Constant  Value=0
  Demux : Demux  Outputs=7
  Display{,1..4} (5 alike) : Display
  EMAT Concatenate : Concatenate  NumInputs=7  Mode=Multidimensional array  ConcatenateDimension=2
  EMAT New : Subsystem
  Matrix Multiply : Product  Multiplication=Matrix(*)
  Product : Product
  Subtract : Sum  Inputs=+-
  Ncf : Outport
  Zf : Outport  Port=2
  Zcl : Outport  Port=3
  Zch : Outport  Port=4
  Wf : Outport  Port=5
  TFth : Outport  Port=6
  TFtl : Outport  Port=7
  wires:
  V1/1 -> Add/2
  V2/1 -> Add1/2
  V3/1 -> Add2/2
  V4/1 -> Add3/2
  V5/1 -> Add4/2
  V6/1 -> Add5/2
  V7/1 -> Add6/2
  Add/1 -> Ncf/1
  Add1/1 -> Zf/1
  Add2/1 -> Zcl/1
  Add3/1 -> Zch/1
  Add5/1 -> TFth/1
  Add6/1 -> TFtl/1
  " LU Inverse"/1(inv(A)) -> Matrix Multiply/1, Display1/1
  Add4/1 -> Wf/1
  EMAT Concatenate/1 -> Display/1, " LU Inverse"/1(A)
  Constant/1 -> Product/1
  Constant1/1 -> Subtract/1
  Matrix Multiply/1 -> Display2/1, Product/2
  Product/1 -> Demux/1, Display4/1
  Demux/1 -> Add/1
  Demux/2 -> Add1/1
  Demux/3 -> Add2/1
  Demux/4 -> Add3/1
  Demux/5 -> Add4/1
  Demux/6 -> Add5/1
  Demux/7 -> Add6/1
  ERS_V1/1 -> EMAT New/1(ERS_V1)
  ERS_V2/1 -> EMAT New/2(ERS_V2)
  ERS_V3/1 -> EMAT New/3(ERS_V3)
  ERS_V4/1 -> EMAT New/4(ERS_V4)
  ERS_V5/1 -> EMAT New/5(ERS_V5)
  ERS_V6/1 -> EMAT New/6(ERS_V6)
  ERS_V7/1 -> EMAT New/7(ERS_V7)
  ERB/1 -> EMAT New/8(ERB), Subtract/2
  DV1/1 -> EMAT New/9(DV1)
  DV2/1 -> EMAT New/10(DV2)
  DV3/1 -> EMAT New/11(DV3)
  DV4/1 -> EMAT New/12(DV4)
  DV5/1 -> EMAT New/13(DV5)
  DV6/1 -> EMAT New/14(DV6)
  DV7/1 -> EMAT New/15(DV7)
  EMAT New/1(EMAT1) -> Display3/1, EMAT Concatenate/1
  EMAT New/2(EMAT2) -> EMAT Concatenate/2
  EMAT New/3(EMAT3) -> EMAT Concatenate/3
  EMAT New/4(EMAT4) -> EMAT Concatenate/4
  EMAT New/5(EMAT5) -> EMAT Concatenate/5
  EMAT New/6(EMAT6) -> EMAT Concatenate/6
  EMAT New/7(EMAT7) -> EMAT Concatenate/7
  Subtract/1 -> Matrix Multiply/2

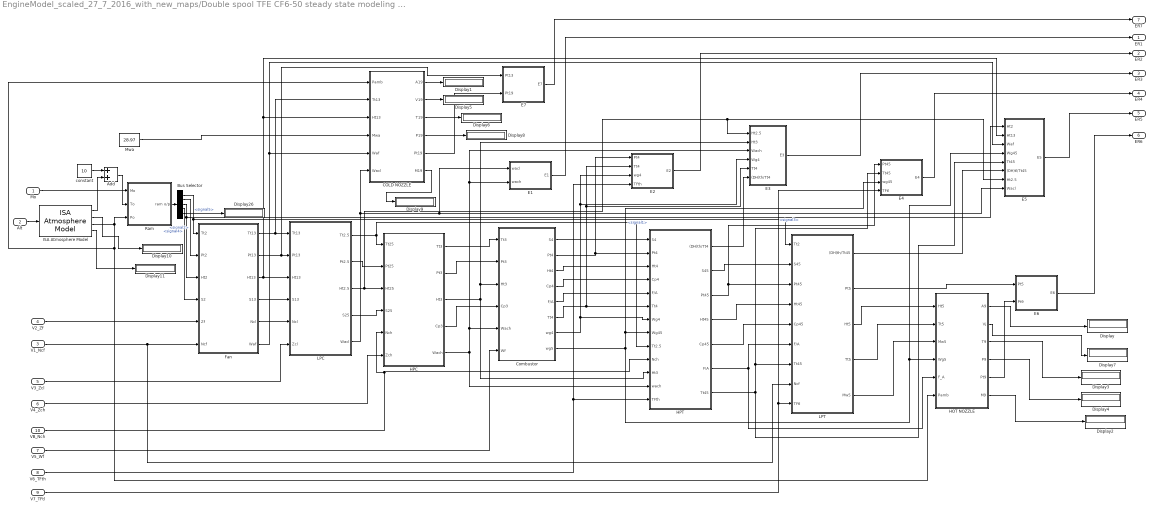
== system EngineModel_scaled_27_7_2016_with_new_maps/Double spool TFE CF6-50 steady state modeling (BOING 747-200)/Error Due to Vs/Error Due To Dv1 ==
  Mo : Inport
  Alt : Inport  Port=2
  V1_Ncf : Inport  Port=3
  V2_Zf : Inport  Port=4
  V3_Zcl : Inport  Port=5
  V4_Zch : Inport  Port=6
  V5_Wf : Inport  Port=7
  V6_TFth : Inport  Port=8
  V7_TFtl : Inport  Port=9
  VB_Nch : Inport  Port=10
  Add : Sum
  Bus Selector : BusSelector  OutputSignals=signal1,signal2,signal3,signal4,signal5
  COLD NOZZLE : Subsystem
  Combustor : Subsystem
  Display{,1..11,26} (13 alike) : Display
  E1 : Subsystem
  E2 : Subsystem
  E3 : Subsystem
  E4 : Subsystem
  E5 : Subsystem
  E6 : Subsystem
  E7 : Subsystem
  Fan : Subsystem
  HOT NOZZLE : Subsystem
  HPC : Subsystem
  HPT : Subsystem
  ISA Atmosphere Model : aerolibatmos2/ISA Atmosphere Model  custom=on  g=9.81  gamma=1.4  R=287  L=0.0065  h_trop=11000  h_strat=20000  rho0=1.225  P0=101325  T0=288  h0=0
  LPC : Subsystem
  LPT : Subsystem
  Mwa : Constant  Value=28.97
  Ram : Subsystem
  constant : Constant  Value=10
  ER1 : Outport
  ER2 : Outport  Port=2
  ER3 : Outport  Port=3
  ER4 : Outport  Port=4
  ER5 : Outport  Port=5
  ER6 : Outport  Port=6
  ER7 : Outport  Port=7
  wires:
  Alt/1 -> ISA Atmosphere Model/1
  Mo/1 -> Ram/1(Mo)
  ISA Atmosphere Model/1 -> Add/2
  Ram/1(ram o/p) -> Bus Selector/1
  ISA Atmosphere Model/3 -> Ram/3(Po), COLD NOZZLE/1(Pamb), HOT NOZZLE/6(Pamb)
  constant/1 -> Add/1
  Add/1 -> Ram/2(To)
  Bus Selector/1 -> Fan/1(Tt2), LPT/1(Tt2)  "<signal1>"
  Bus Selector/2 -> Fan/2(Pt2)  "<signal2>"
  Fan/1(Tt13) -> LPC/1(Tt13), COLD NOZZLE/2(Tt13)
  Fan/2(Pt13) -> E7/1(Pt13), LPC/2(Pt13)
  LPC/1(Tt2.5) -> HPC/1(Tt25), HPT/9(Tt2.5)
  LPC/2(Pt2.5) -> HPC/2(Pt25)
  HPC/1(Tt3) -> Combustor/1(Tt3)
  HPC/2(Pt3) -> Combustor/2(Pt3)
  HPC/3(Ht3) -> Combustor/3(Ht3), E3/2(Ht3), HPT/11(Ht3)
  Combustor/2(Pt4) -> E2/1(Pt4), HPT/2(Pt4)
  Combustor/4(Cp4) -> HPT/4(Cp4)
  Combustor/5(F/A) -> HPT/5(F/A)
  Combustor/6(Tt4) -> E2/2(Tt4), E3/5(Tt4), HPT/6(Tt4)
  LPT/3(Ht5) -> HOT NOZZLE/1(Ht5)
  LPT/4(Tt5) -> HOT NOZZLE/2(Tt5)
  V2_Zf/1 -> Fan/5(Zf)
  V1_Ncf/1 -> LPT/8(Ncf), Fan/6(Ncf)
  V3_Zcl/1 -> LPC/6(Zcl)
  V4_Zch/1 -> HPC/6(Zch)
  VB_Nch/1 -> HPT/10(Nch), HPC/5(Nch)
  V5_Wf/1 -> Combustor/6(Wf)
  V6_TFth/1 -> E2/4(TFth), HPT/13(TFth)
  Combustor/7(wg4) -> E2/3(wg4), E3/4(Wg4), HPT/7(Wg4)
  LPT/5(Mw5) -> HOT NOZZLE/3(Mw5)
  Fan/3(Ht13) -> COLD NOZZLE/3(Ht13), E5/2(Ht13), LPC/3(Ht13)
  Mwa/1 -> COLD NOZZLE/4(Mwa)
  Fan/6(Waf) -> E5/3(Waf), COLD NOZZLE/5(Waf)
  LPC/5(Wacl) -> COLD NOZZLE/6(Wacl), E1/1(wacl), E5/8(Wacl)
  COLD NOZZLE/5(Pt19) -> E7/2(Pt19)
  LPC/3(Ht2.5) -> HPC/3(Ht25), E3/1(Ht2.5), E5/7(Ht2.5)
  LPT/2(Pt5) -> E6/1(Pt5)
  HOT NOZZLE/5(Pt9) -> E6/2(Pt9)
  LPT/1((DH)th/Tt45) -> E5/6((DH)tl/Tt45)
  Combustor/8(wg5) -> E4/3(wg45), HPT/8(Wg45), E5/4(Wg45), HOT NOZZLE/4(Wg5)
  Combustor/3(Ht4) -> HPT/3(Ht4)
  Combustor/1(S4) -> HPT/1(S4)
  HOT NOZZLE/1(A9) -> Display/1
  HOT NOZZLE/2(Vj) -> Display7/1
  HOT NOZZLE/3(T9) -> Display3/1
  HOT NOZZLE/4(P9) -> Display4/1
  HOT NOZZLE/6(M9) -> Display2/1
  Bus Selector/3 -> Fan/3(Ht2), E5/1(Ht2)  "<signal3>"
  Bus Selector/4 -> Fan/4(S2)  "<signal4>"
  Fan/5(Ncl) -> LPC/5(Ncl)
  Fan/4(S13) -> LPC/4(S13)
  LPC/4(S25) -> HPC/4(S25)
  HPC/5(Wach) -> Combustor/5(Wach), E3/3(Wach), E1/2(wach), HPT/12(wach)
  HPT/2(S45) -> LPT/2(S45)
  HPT/3(Pt45) -> E4/1(Pt45), LPT/3(Pt45)
  HPT/4(Ht45) -> LPT/4(Ht45)
  HPT/5(Cp45) -> LPT/5(Cp45)
  HPT/7(Tt45) -> LPT/7(Tt45), E4/2(Tt45), E5/5(Tt45)
  HPT/6(F\A) -> LPT/6(F/A), HOT NOZZLE/5(F_A)
  V7_TFtl/1 -> LPT/9(TFtl), E4/4(TFtl)
  HPT/1((DH)th/Tt4) -> E3/6((DH)th/Tt4)
  E6/1(E6) -> ER6/1
  E5/1(E5) -> ER5/1
  E4/1(E4) -> ER4/1
  E3/1(E3) -> ER3/1
  E2/1(E2) -> ER2/1
  E1/1(E1) -> ER1/1
  E7/1(E7) -> ER7/1
  HPC/4(Cp3) -> Combustor/4(Cp3)
  Bus Selector/5 -> Display26/1  "<signal5>"
  COLD NOZZLE/1(A19) -> Display1/1
  COLD NOZZLE/2(V19) -> Display5/1
  COLD NOZZLE/3(T19) -> Display6/1
  COLD NOZZLE/4(P19) -> Display8/1
  COLD NOZZLE/6(M19) -> Display9/1
  ISA Atmosphere Model/2 -> Display10/1
  ISA Atmosphere Model/4 -> Display11/1

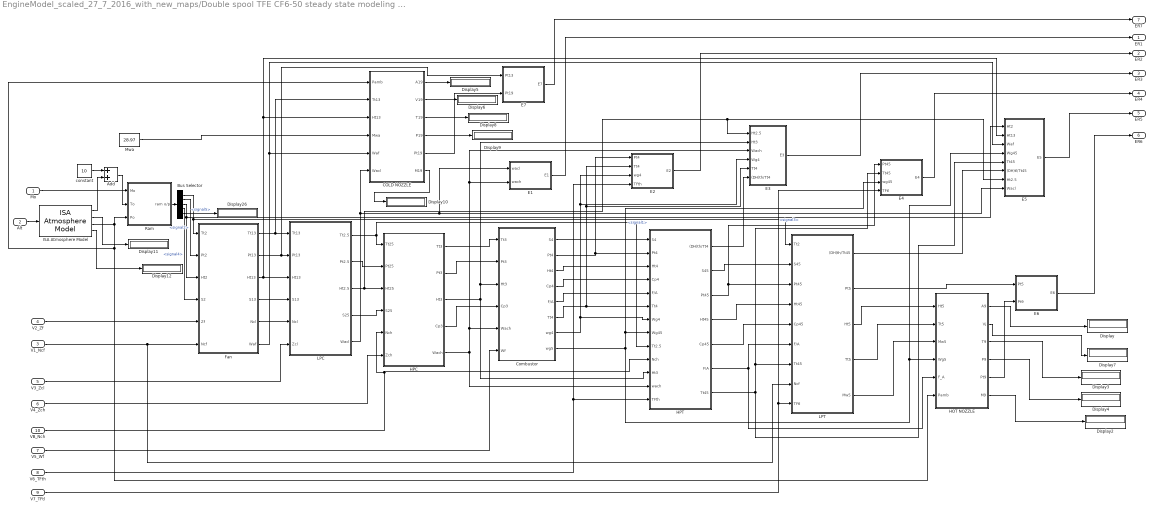
== system EngineModel_scaled_27_7_2016_with_new_maps/Double spool TFE CF6-50 steady state modeling (BOING 747-200)/Error Due to Vs/Error Due To Dv2 ==
  Mo : Inport
  Alt : Inport  Port=2
  V1_Ncf : Inport  Port=3
  V2_Zf : Inport  Port=4
  V3_Zcl : Inport  Port=5
  V4_Zch : Inport  Port=6
  V5_Wf : Inport  Port=7
  V6_TFth : Inport  Port=8
  V7_TFtl : Inport  Port=9
  VB_Nch : Inport  Port=10
  Add : Sum
  Bus Selector : BusSelector  OutputSignals=signal1,signal2,signal3,signal4,signal5
  COLD NOZZLE : Subsystem
  Combustor : Subsystem
  Display{,2..12,26} (13 alike) : Display
  E1 : Subsystem
  E2 : Subsystem
  E3 : Subsystem
  E4 : Subsystem
  E5 : Subsystem
  E6 : Subsystem
  E7 : Subsystem
  Fan : Subsystem
  HOT NOZZLE : Subsystem
  HPC : Subsystem
  HPT : Subsystem
  ISA Atmosphere Model : aerolibatmos2/ISA Atmosphere Model  custom=on  g=9.81  gamma=1.4  R=287  L=0.0065  h_trop=11000  h_strat=20000  rho0=1.225  P0=101325  T0=288  h0=0
  LPC : Subsystem
  LPT : Subsystem
  Mwa : Constant  Value=28.97
  Ram : Subsystem
  constant : Constant  Value=10
  ER1 : Outport
  ER2 : Outport  Port=2
  ER3 : Outport  Port=3
  ER4 : Outport  Port=4
  ER5 : Outport  Port=5
  ER6 : Outport  Port=6
  ER7 : Outport  Port=7
  wires:
  HPC/4(Cp3) -> Combustor/4(Cp3)
  E7/1(E7) -> ER7/1
  E1/1(E1) -> ER1/1
  E2/1(E2) -> ER2/1
  E3/1(E3) -> ER3/1
  E4/1(E4) -> ER4/1
  E5/1(E5) -> ER5/1
  E6/1(E6) -> ER6/1
  HPT/1((DH)th/Tt4) -> E3/6((DH)th/Tt4)
  V7_TFtl/1 -> E4/4(TFtl), LPT/9(TFtl)
  HPT/6(F\A) -> HOT NOZZLE/5(F_A), LPT/6(F/A)
  HPT/7(Tt45) -> E5/5(Tt45), E4/2(Tt45), LPT/7(Tt45)
  HPT/5(Cp45) -> LPT/5(Cp45)
  HPT/4(Ht45) -> LPT/4(Ht45)
  HPT/3(Pt45) -> LPT/3(Pt45), E4/1(Pt45)
  HPT/2(S45) -> LPT/2(S45)
  HPC/5(Wach) -> HPT/12(wach), E1/2(wach), E3/3(Wach), Combustor/5(Wach)
  LPC/4(S25) -> HPC/4(S25)
  Fan/4(S13) -> LPC/4(S13)
  Fan/5(Ncl) -> LPC/5(Ncl)
  Bus Selector/4 -> Fan/4(S2)  "<signal4>"
  Bus Selector/3 -> E5/1(Ht2), Fan/3(Ht2)  "<signal3>"
  HOT NOZZLE/6(M9) -> Display2/1
  HOT NOZZLE/4(P9) -> Display4/1
  HOT NOZZLE/3(T9) -> Display3/1
  HOT NOZZLE/2(Vj) -> Display7/1
  HOT NOZZLE/1(A9) -> Display/1
  Combustor/1(S4) -> HPT/1(S4)
  Combustor/3(Ht4) -> HPT/3(Ht4)
  Combustor/8(wg5) -> HOT NOZZLE/4(Wg5), E5/4(Wg45), HPT/8(Wg45), E4/3(wg45)
  LPT/1((DH)th/Tt45) -> E5/6((DH)tl/Tt45)
  HOT NOZZLE/5(Pt9) -> E6/2(Pt9)
  LPT/2(Pt5) -> E6/1(Pt5)
  LPC/3(Ht2.5) -> E5/7(Ht2.5), E3/1(Ht2.5), HPC/3(Ht25)
  COLD NOZZLE/5(Pt19) -> E7/2(Pt19)
  LPC/5(Wacl) -> E5/8(Wacl), E1/1(wacl), COLD NOZZLE/6(Wacl)
  Fan/6(Waf) -> COLD NOZZLE/5(Waf), E5/3(Waf)
  Mwa/1 -> COLD NOZZLE/4(Mwa)
  Fan/3(Ht13) -> LPC/3(Ht13), E5/2(Ht13), COLD NOZZLE/3(Ht13)
  LPT/5(Mw5) -> HOT NOZZLE/3(Mw5)
  Combustor/7(wg4) -> HPT/7(Wg4), E3/4(Wg4), E2/3(wg4)
  V6_TFth/1 -> HPT/13(TFth), E2/4(TFth)
  V5_Wf/1 -> Combustor/6(Wf)
  VB_Nch/1 -> HPC/5(Nch), HPT/10(Nch)
  V4_Zch/1 -> HPC/6(Zch)
  V3_Zcl/1 -> LPC/6(Zcl)
  V1_Ncf/1 -> Fan/6(Ncf), LPT/8(Ncf)
  V2_Zf/1 -> Fan/5(Zf)
  LPT/4(Tt5) -> HOT NOZZLE/2(Tt5)
  LPT/3(Ht5) -> HOT NOZZLE/1(Ht5)
  Combustor/6(Tt4) -> HPT/6(Tt4), E3/5(Tt4), E2/2(Tt4)
  Combustor/5(F/A) -> HPT/5(F/A)
  Combustor/4(Cp4) -> HPT/4(Cp4)
  Combustor/2(Pt4) -> HPT/2(Pt4), E2/1(Pt4)
  HPC/3(Ht3) -> HPT/11(Ht3), E3/2(Ht3), Combustor/3(Ht3)
  HPC/2(Pt3) -> Combustor/2(Pt3)
  HPC/1(Tt3) -> Combustor/1(Tt3)
  LPC/2(Pt2.5) -> HPC/2(Pt25)
  LPC/1(Tt2.5) -> HPT/9(Tt2.5), HPC/1(Tt25)
  Fan/2(Pt13) -> LPC/2(Pt13), E7/1(Pt13)
  Fan/1(Tt13) -> COLD NOZZLE/2(Tt13), LPC/1(Tt13)
  Bus Selector/2 -> Fan/2(Pt2)  "<signal2>"
  Bus Selector/1 -> LPT/1(Tt2), Fan/1(Tt2)  "<signal1>"
  Add/1 -> Ram/2(To)
  constant/1 -> Add/1
  ISA Atmosphere Model/3 -> HOT NOZZLE/6(Pamb), COLD NOZZLE/1(Pamb), Ram/3(Po)
  Ram/1(ram o/p) -> Bus Selector/1
  ISA Atmosphere Model/1 -> Add/2
  Mo/1 -> Ram/1(Mo)
  Alt/1 -> ISA Atmosphere Model/1
  Bus Selector/5 -> Display26/1  "<signal5>"
  COLD NOZZLE/1(A19) -> Display5/1
  COLD NOZZLE/2(V19) -> Display6/1
  COLD NOZZLE/3(T19) -> Display8/1
  COLD NOZZLE/4(P19) -> Display9/1
  COLD NOZZLE/6(M19) -> Display10/1
  ISA Atmosphere Model/2 -> Display11/1
  ISA Atmosphere Model/4 -> Display12/1

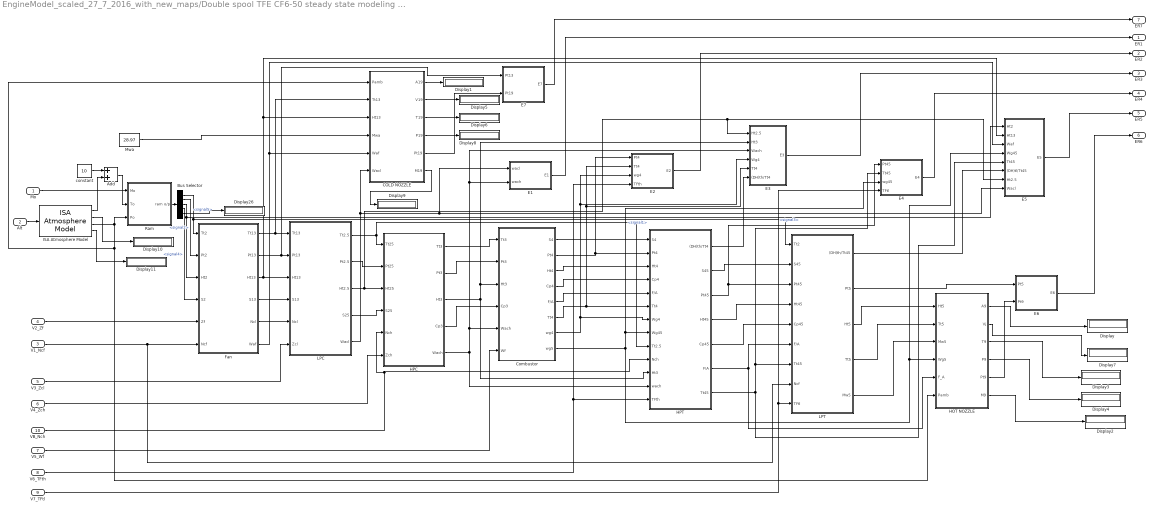
== system EngineModel_scaled_27_7_2016_with_new_maps/Double spool TFE CF6-50 steady state modeling (BOING 747-200)/Error Due to Vs/Error Due To Dv3 ==
  Mo : Inport
  Alt : Inport  Port=2
  V1_Ncf : Inport  Port=3
  V2_Zf : Inport  Port=4
  V3_Zcl : Inport  Port=5
  V4_Zch : Inport  Port=6
  V5_Wf : Inport  Port=7
  V6_TFth : Inport  Port=8
  V7_TFtl : Inport  Port=9
  VB_Nch : Inport  Port=10
  Add : Sum
  Bus Selector : BusSelector  OutputSignals=signal1,signal2,signal3,signal4,signal5
  COLD NOZZLE : Subsystem
  Combustor : Subsystem
  Display{,1..11,26} (13 alike) : Display
  E1 : Subsystem
  E2 : Subsystem
  E3 : Subsystem
  E4 : Subsystem
  E5 : Subsystem
  E6 : Subsystem
  E7 : Subsystem
  Fan : Subsystem
  HOT NOZZLE : Subsystem
  HPC : Subsystem
  HPT : Subsystem
  ISA Atmosphere Model : aerolibatmos2/ISA Atmosphere Model  custom=on  g=9.81  gamma=1.4  R=287  L=0.0065  h_trop=11000  h_strat=20000  rho0=1.225  P0=101325  T0=288  h0=0
  LPC : Subsystem
  LPT : Subsystem
  Mwa : Constant  Value=28.97
  Ram : Subsystem
  constant : Constant  Value=10
  ER1 : Outport
  ER2 : Outport  Port=2
  ER3 : Outport  Port=3
  ER4 : Outport  Port=4
  ER5 : Outport  Port=5
  ER6 : Outport  Port=6
  ER7 : Outport  Port=7
  wires:
  Alt/1 -> ISA Atmosphere Model/1
  Mo/1 -> Ram/1(Mo)
  ISA Atmosphere Model/1 -> Add/2
  Ram/1(ram o/p) -> Bus Selector/1
  ISA Atmosphere Model/3 -> Ram/3(Po), COLD NOZZLE/1(Pamb), HOT NOZZLE/6(Pamb)
  constant/1 -> Add/1
  Add/1 -> Ram/2(To)
  Bus Selector/1 -> Fan/1(Tt2), LPT/1(Tt2)  "<signal1>"
  Bus Selector/2 -> Fan/2(Pt2)  "<signal2>"
  Fan/1(Tt13) -> LPC/1(Tt13), COLD NOZZLE/2(Tt13)
  Fan/2(Pt13) -> E7/1(Pt13), LPC/2(Pt13)
  LPC/1(Tt2.5) -> HPC/1(Tt25), HPT/9(Tt2.5)
  LPC/2(Pt2.5) -> HPC/2(Pt25)
  HPC/1(Tt3) -> Combustor/1(Tt3)
  HPC/2(Pt3) -> Combustor/2(Pt3)
  HPC/3(Ht3) -> Combustor/3(Ht3), E3/2(Ht3), HPT/11(Ht3)
  Combustor/2(Pt4) -> E2/1(Pt4), HPT/2(Pt4)
  Combustor/4(Cp4) -> HPT/4(Cp4)
  Combustor/5(F/A) -> HPT/5(F/A)
  Combustor/6(Tt4) -> E2/2(Tt4), E3/5(Tt4), HPT/6(Tt4)
  LPT/3(Ht5) -> HOT NOZZLE/1(Ht5)
  LPT/4(Tt5) -> HOT NOZZLE/2(Tt5)
  V2_Zf/1 -> Fan/5(Zf)
  V1_Ncf/1 -> LPT/8(Ncf), Fan/6(Ncf)
  V3_Zcl/1 -> LPC/6(Zcl)
  V4_Zch/1 -> HPC/6(Zch)
  VB_Nch/1 -> HPT/10(Nch), HPC/5(Nch)
  V5_Wf/1 -> Combustor/6(Wf)
  V6_TFth/1 -> E2/4(TFth), HPT/13(TFth)
  Combustor/7(wg4) -> E2/3(wg4), E3/4(Wg4), HPT/7(Wg4)
  LPT/5(Mw5) -> HOT NOZZLE/3(Mw5)
  Fan/3(Ht13) -> COLD NOZZLE/3(Ht13), E5/2(Ht13), LPC/3(Ht13)
  Mwa/1 -> COLD NOZZLE/4(Mwa)
  Fan/6(Waf) -> E5/3(Waf), COLD NOZZLE/5(Waf)
  LPC/5(Wacl) -> COLD NOZZLE/6(Wacl), E1/1(wacl), E5/8(Wacl)
  COLD NOZZLE/5(Pt19) -> E7/2(Pt19)
  LPC/3(Ht2.5) -> HPC/3(Ht25), E3/1(Ht2.5), E5/7(Ht2.5)
  LPT/2(Pt5) -> E6/1(Pt5)
  HOT NOZZLE/5(Pt9) -> E6/2(Pt9)
  LPT/1((DH)th/Tt45) -> E5/6((DH)tl/Tt45)
  Combustor/8(wg5) -> E4/3(wg45), HPT/8(Wg45), E5/4(Wg45), HOT NOZZLE/4(Wg5)
  Combustor/3(Ht4) -> HPT/3(Ht4)
  Combustor/1(S4) -> HPT/1(S4)
  HOT NOZZLE/1(A9) -> Display/1
  HOT NOZZLE/2(Vj) -> Display7/1
  HOT NOZZLE/3(T9) -> Display3/1
  HOT NOZZLE/4(P9) -> Display4/1
  HOT NOZZLE/6(M9) -> Display2/1
  Bus Selector/3 -> Fan/3(Ht2), E5/1(Ht2)  "<signal3>"
  Bus Selector/4 -> Fan/4(S2)  "<signal4>"
  Fan/5(Ncl) -> LPC/5(Ncl)
  Fan/4(S13) -> LPC/4(S13)
  LPC/4(S25) -> HPC/4(S25)
  HPC/5(Wach) -> Combustor/5(Wach), E3/3(Wach), E1/2(wach), HPT/12(wach)
  HPT/2(S45) -> LPT/2(S45)
  HPT/3(Pt45) -> E4/1(Pt45), LPT/3(Pt45)
  HPT/4(Ht45) -> LPT/4(Ht45)
  HPT/5(Cp45) -> LPT/5(Cp45)
  HPT/7(Tt45) -> LPT/7(Tt45), E4/2(Tt45), E5/5(Tt45)
  HPT/6(F\A) -> LPT/6(F/A), HOT NOZZLE/5(F_A)
  V7_TFtl/1 -> LPT/9(TFtl), E4/4(TFtl)
  HPT/1((DH)th/Tt4) -> E3/6((DH)th/Tt4)
  E6/1(E6) -> ER6/1
  E5/1(E5) -> ER5/1
  E4/1(E4) -> ER4/1
  E3/1(E3) -> ER3/1
  E2/1(E2) -> ER2/1
  E1/1(E1) -> ER1/1
  E7/1(E7) -> ER7/1
  HPC/4(Cp3) -> Combustor/4(Cp3)
  Bus Selector/5 -> Display26/1  "<signal5>"
  COLD NOZZLE/1(A19) -> Display1/1
  COLD NOZZLE/2(V19) -> Display5/1
  COLD NOZZLE/3(T19) -> Display6/1
  COLD NOZZLE/4(P19) -> Display8/1
  COLD NOZZLE/6(M19) -> Display9/1
  ISA Atmosphere Model/2 -> Display10/1
  ISA Atmosphere Model/4 -> Display11/1

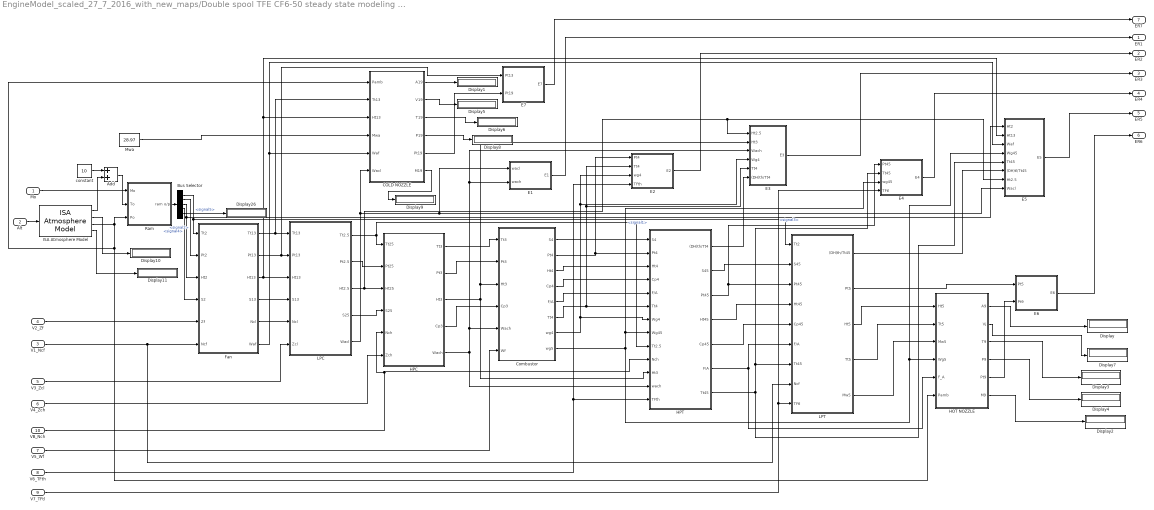
== system EngineModel_scaled_27_7_2016_with_new_maps/Double spool TFE CF6-50 steady state modeling (BOING 747-200)/Error Due to Vs/Error Due To Dv4 ==
  Mo : Inport
  Alt : Inport  Port=2
  V1_Ncf : Inport  Port=3
  V2_Zf : Inport  Port=4
  V3_Zcl : Inport  Port=5
  V4_Zch : Inport  Port=6
  V5_Wf : Inport  Port=7
  V6_TFth : Inport  Port=8
  V7_TFtl : Inport  Port=9
  VB_Nch : Inport  Port=10
  Add : Sum
  Bus Selector : BusSelector  OutputSignals=signal1,signal2,signal3,signal4,signal5
  COLD NOZZLE : Subsystem
  Combustor : Subsystem
  Display{,1..11,26} (13 alike) : Display
  E1 : Subsystem
  E2 : Subsystem
  E3 : Subsystem
  E4 : Subsystem
  E5 : Subsystem
  E6 : Subsystem
  E7 : Subsystem
  Fan : Subsystem
  HOT NOZZLE : Subsystem
  HPC : Subsystem
  HPT : Subsystem
  ISA Atmosphere Model : aerolibatmos2/ISA Atmosphere Model  custom=on  g=9.81  gamma=1.4  R=287  L=0.0065  h_trop=11000  h_strat=20000  rho0=1.225  P0=101325  T0=288  h0=0
  LPC : Subsystem
  LPT : Subsystem
  Mwa : Constant  Value=28.97
  Ram : Subsystem
  constant : Constant  Value=10
  ER1 : Outport
  ER2 : Outport  Port=2
  ER3 : Outport  Port=3
  ER4 : Outport  Port=4
  ER5 : Outport  Port=5
  ER6 : Outport  Port=6
  ER7 : Outport  Port=7
  wires:
  HPC/4(Cp3) -> Combustor/4(Cp3)
  E7/1(E7) -> ER7/1
  E1/1(E1) -> ER1/1
  E2/1(E2) -> ER2/1
  E3/1(E3) -> ER3/1
  E4/1(E4) -> ER4/1
  E5/1(E5) -> ER5/1
  E6/1(E6) -> ER6/1
  HPT/1((DH)th/Tt4) -> E3/6((DH)th/Tt4)
  V7_TFtl/1 -> E4/4(TFtl), LPT/9(TFtl)
  HPT/6(F\A) -> HOT NOZZLE/5(F_A), LPT/6(F/A)
  HPT/7(Tt45) -> E5/5(Tt45), E4/2(Tt45), LPT/7(Tt45)
  HPT/5(Cp45) -> LPT/5(Cp45)
  HPT/4(Ht45) -> LPT/4(Ht45)
  HPT/3(Pt45) -> LPT/3(Pt45), E4/1(Pt45)
  HPT/2(S45) -> LPT/2(S45)
  HPC/5(Wach) -> HPT/12(wach), E1/2(wach), E3/3(Wach), Combustor/5(Wach)
  LPC/4(S25) -> HPC/4(S25)
  Fan/4(S13) -> LPC/4(S13)
  Fan/5(Ncl) -> LPC/5(Ncl)
  Bus Selector/4 -> Fan/4(S2)  "<signal4>"
  Bus Selector/3 -> E5/1(Ht2), Fan/3(Ht2)  "<signal3>"
  HOT NOZZLE/6(M9) -> Display2/1
  HOT NOZZLE/4(P9) -> Display4/1
  HOT NOZZLE/3(T9) -> Display3/1
  HOT NOZZLE/2(Vj) -> Display7/1
  HOT NOZZLE/1(A9) -> Display/1
  Combustor/1(S4) -> HPT/1(S4)
  Combustor/3(Ht4) -> HPT/3(Ht4)
  Combustor/8(wg5) -> HOT NOZZLE/4(Wg5), E5/4(Wg45), HPT/8(Wg45), E4/3(wg45)
  LPT/1((DH)th/Tt45) -> E5/6((DH)tl/Tt45)
  HOT NOZZLE/5(Pt9) -> E6/2(Pt9)
  LPT/2(Pt5) -> E6/1(Pt5)
  LPC/3(Ht2.5) -> E5/7(Ht2.5), E3/1(Ht2.5), HPC/3(Ht25)
  COLD NOZZLE/5(Pt19) -> E7/2(Pt19)
  LPC/5(Wacl) -> E5/8(Wacl), E1/1(wacl), COLD NOZZLE/6(Wacl)
  Fan/6(Waf) -> COLD NOZZLE/5(Waf), E5/3(Waf)
  Mwa/1 -> COLD NOZZLE/4(Mwa)
  Fan/3(Ht13) -> LPC/3(Ht13), E5/2(Ht13), COLD NOZZLE/3(Ht13)
  LPT/5(Mw5) -> HOT NOZZLE/3(Mw5)
  Combustor/7(wg4) -> HPT/7(Wg4), E3/4(Wg4), E2/3(wg4)
  V6_TFth/1 -> HPT/13(TFth), E2/4(TFth)
  V5_Wf/1 -> Combustor/6(Wf)
  VB_Nch/1 -> HPC/5(Nch), HPT/10(Nch)
  V4_Zch/1 -> HPC/6(Zch)
  V3_Zcl/1 -> LPC/6(Zcl)
  V1_Ncf/1 -> Fan/6(Ncf), LPT/8(Ncf)
  V2_Zf/1 -> Fan/5(Zf)
  LPT/4(Tt5) -> HOT NOZZLE/2(Tt5)
  LPT/3(Ht5) -> HOT NOZZLE/1(Ht5)
  Combustor/6(Tt4) -> HPT/6(Tt4), E3/5(Tt4), E2/2(Tt4)
  Combustor/5(F/A) -> HPT/5(F/A)
  Combustor/4(Cp4) -> HPT/4(Cp4)
  Combustor/2(Pt4) -> HPT/2(Pt4), E2/1(Pt4)
  HPC/3(Ht3) -> HPT/11(Ht3), E3/2(Ht3), Combustor/3(Ht3)
  HPC/2(Pt3) -> Combustor/2(Pt3)
  HPC/1(Tt3) -> Combustor/1(Tt3)
  LPC/2(Pt2.5) -> HPC/2(Pt25)
  LPC/1(Tt2.5) -> HPT/9(Tt2.5), HPC/1(Tt25)
  Fan/2(Pt13) -> LPC/2(Pt13), E7/1(Pt13)
  Fan/1(Tt13) -> COLD NOZZLE/2(Tt13), LPC/1(Tt13)
  Bus Selector/2 -> Fan/2(Pt2)  "<signal2>"
  Bus Selector/1 -> LPT/1(Tt2), Fan/1(Tt2)  "<signal1>"
  Add/1 -> Ram/2(To)
  constant/1 -> Add/1
  ISA Atmosphere Model/3 -> HOT NOZZLE/6(Pamb), COLD NOZZLE/1(Pamb), Ram/3(Po)
  Ram/1(ram o/p) -> Bus Selector/1
  ISA Atmosphere Model/1 -> Add/2
  Mo/1 -> Ram/1(Mo)
  Alt/1 -> ISA Atmosphere Model/1
  Bus Selector/5 -> Display26/1  "<signal5>"
  COLD NOZZLE/1(A19) -> Display1/1
  COLD NOZZLE/2(V19) -> Display5/1
  COLD NOZZLE/3(T19) -> Display6/1
  COLD NOZZLE/4(P19) -> Display8/1
  COLD NOZZLE/6(M19) -> Display9/1
  ISA Atmosphere Model/2 -> Display10/1
  ISA Atmosphere Model/4 -> Display11/1
